simulink model "sl_subsys_for2"  (Simulink 7.6)
settings: Solver=FixedStepDiscrete  StartTime=0.0  StopTime=10.0  FixedStep=1  RelTol=1e-3
Description:
  | For subsystem example with assignment block
settings Model: Creator=The MathWorks Inc.  ExtModeAutoUpdateStatusClock=off
settings OptimizationCC: BooleanDataType=off  InitFltsAndDblsToZero=on
settings DebuggingCC: SaveWithParameterizedLinksMsg=none  SignalResolutionControl=TryResolveAllWithWarning  SolverPrmCheckMsg=none  MultiTaskDSMMsg=warning  MultiTaskCondExecSysMsg=none
settings HardwareCC: TargetUnknown=on
settings RTWCC: IncludeERTFirstTime=on
settings CodeAppCC: CustomSymbolStrFcn=$F$N$M
settings GRTTargetCC: TargetFcnLib=ansi_tfl_tmw.mat

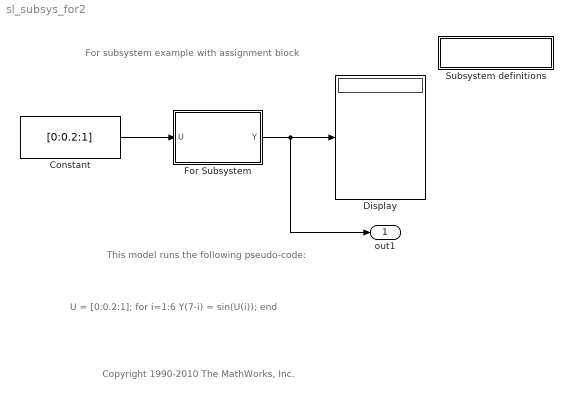
== system sl_subsys_for2 ==
  note: This model runs the following pseudo-code:
  note: U = [0:0.2:1];
      |       for i=1:6
      |                            Y(7-i) = sin(U(i));
      | end
  note: For subsystem example with assignment block
  note: Copyright 1990-2010 The MathWorks, Inc.
  " Subsystem definitions" : Subsystem
      settings: OpenFcn=helpview([matlabroot,'/toolbox/simulink/simdemos/simfeatures/html/sl_subsys_definitions.html']);
      mask Display: disp('Subsystem\ndefinitions')
  Constant : Constant  Value=[0:0.2:1]
  Display : Display
  For Subsystem : Subsystem  TreatAsAtomicUnit=on
  out1 : Outport
  wires:
  Constant/1 -> For Subsystem/1(U)
  For Subsystem/1(Y) -> Display/1, out1/1

== system sl_subsys_for2/ Subsystem definitions ==

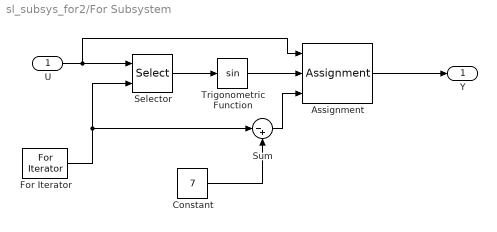
== system sl_subsys_for2/For Subsystem ==
  U : Inport
  Assignment : Assignment  IndexOptions=Index vector (port)  Indices=1  OutputSizes=[1 1]
  Constant : Constant  Value=7
  For Iterator : ForIterator  ResetStates=reset  IterationLimit=6  IterationVariableDataType=double
  Selector : Selector  IndexOptions=Index vector (port)  Indices=[1 3]  OutputSizes=1
  Sum : Sum  Inputs=|-+  SaturateOnIntegerOverflow=on  InputSameDT=on  OutDataTypeStr=Inherit: Same as first input
  Trigonometric Function : Trigonometry
  Y : Outport
  wires:
  For Iterator/1 -> Selector/2, Sum/1
  U/1 -> Selector/1, Assignment/1
  Selector/1 -> Trigonometric Function/1
  Assignment/1 -> Y/1
  Trigonometric Function/1 -> Assignment/2
  Constant/1 -> Sum/2
  Sum/1 -> Assignment/3
